simulink model "F429_OneADC"  (R2018b)
settings: Solver=FixedStepDiscrete  StartTime=0.0  StopTime=10.0  FixedStep=0.016  RelTol=1e-3  EnableMultiTasking=on
libraries: ADC_Lib x1, STM32_Config_Lib x1, TIMERS_Lib x1, USART_Lib x1
settings Model: Creator=reynaudp  LastModifiedBy=fenard1
settings DataIOCC: LimitDataPoints=on  SaveFormat=Array
settings OptimizationCC: DefaultParameterBehavior=Inlined  LifeSpan=1
settings DebuggingCC: UnderspecifiedInitializationDetection=Classic  MergeDetectMultiDrivingBlocksExec=none  SolverPrmCheckMsg=warning  UniqueDataStoreMsg=error  AllowSymbolicDim=off  StrictBusMsg=ErrorOnBusTreatedAsVector  SFUnexpectedBacktrackingDiag=warning  SFNoUnconditionalDefaultTransitionDiag=warning  SFExecutionAtInitializationDiag=none
settings HardwareCC: ProdBitPerPointer=32  ProdBitPerSizeT=32  ProdBitPerPtrDiffT=32  ProdLargestAtomicInteger=Integer  ProdWordSize=32  ProdHWDeviceType=STMicroelectronics->STM32 32-bit Cortex-M  TargetBitPerPointer=64  TargetBitPerSizeT=64  TargetBitPerPtrDiffT=64  TargetLongLongMode=on  TargetIntDivRoundTo=Zero  TargetEndianess=LittleEndian  TargetWordSize=64  TargetHWDeviceType=MATLAB Host  ProdEqTarget=off
settings ModelReferenceCC: PropagateSignalLabelsOutOfModel=off
settings SFSimCC: SimUseLocalCustomCode=off  CompileTimeRecursionLimit=0  EnableRuntimeRecursion=off  MATLABDynamicMemAlloc=off
settings RTWCC: SystemTargetFile=stm32.tlc  TemplateMakefile=stm32.tmf  Description=stm32 (Embedded Target)  RTWUseLocalCustomCode=off  IncludeHyperlinkInReport=on
settings CodeAppCC: IgnoreCustomStorageClasses=off  CustomSymbolStrType=$N$R$M  SimulinkBlockComments=off
settings STFCustomTargetCC: ParMdlRefBuildCompliant=on  IncludeMdlTerminateFcn=off  CombineOutputUpdateFcns=on  ERTCustomFileBanners=on  SupportComplex=off  SupportContinuousTime=off  SupportNonInlinedSFcns=off  RemoveResetFunc=on  MATLABClassNameForMDSCustomization=Simulink.SoftwareTarget.ERTCustomization  SystemTargetFile=stm32.tlc
settings ERTTargetCC: MultiwordLength=2048  CompOptLevelCompliant=off  ConcurrentExecutionCompliant=off  IncludeMdlTerminateFcn=off  SupportComplex=off  ModelStepFunctionPrototypeControlCompliant=off  CPPClassGenCompliant=off  UseToolchainInfoCompliant=off  ERTSrcFileBannerTemplate=sourceFileTemplate.cgt  ERTHdrFileBannerTemplate=sourceFileTemplate.cgt  ERTDataSrcFileTemplate=sourceFileTemplate.cgt  ERTDataHdrFileTemplate=sourceFileTemplate.cgt  ERTCustomFileTemplate=customRoutineProcess.tlc  ConvertIfToSwitch=off  SuppressUnreachableDefaultCases=off
settings ConfigComp: CovMetricSettings=dw  CovHtmlReporting=on  CovSaveCumulativeToWorkspaceVar=on  CovSaveSingleToWorkspaceVar=on  CovExternalEMLEnable=off  CovSFcnEnable=off

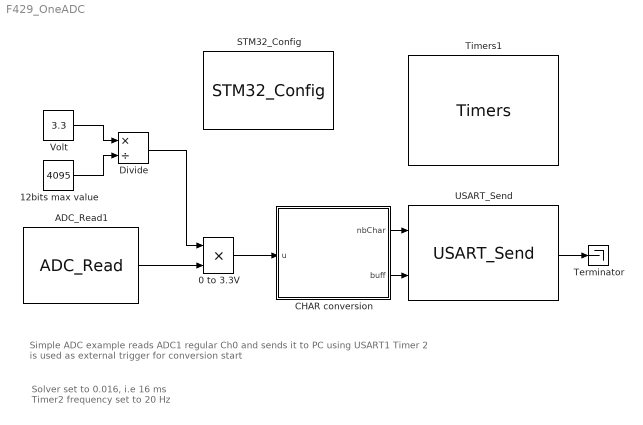
== system F429_OneADC ==
  note: Solver set to 0.016, i.e 16 ms
      | Timer2 frequency set to 20 Hz
  note: Simple ADC example reads ADC1 regular Ch0 and sends it to PC using USART1
      | Timer 2 is used as external trigger for conversion start
  0 to 3.3V : Product  RndMeth=Zero
  12bits max value : Constant  Value=4095
  ADC_Read1 : ADC_Lib/ADC_Read  ADC_Name=ADC1  ADC_Ch0=on  ADC_Ch1=off  ADC_Ch2=off  ADC_Ch3=off  ADC_Ch4=off  ADC_Ch5=off  ADC_Ch6=off  ADC_Ch7=off  ADC_Ch8=off  ADC_Ch9=off  ADC_Ch10=off  ADC_Ch11=off  ADC_Ch12=off  ADC_Ch13=off  ADC_Ch14=off  ADC_Ch15=off  ADC_Ch16=off  ADC_Ch17=off  ADC_Ch18=off  RgRk1=on  RgRk2=off  RgRk3=off  RgRk4=off  RgRk1_Ch=Ch0_r1  RgRk2_Ch=off  RgRk3_Ch=off  RgRk4_Ch=off  RgRk5=off  RgRk6=off  RgRk7=off  RgRk8=off  RgRk5_Ch=off  RgRk6_Ch=off  RgRk7_Ch=off  RgRk8_Ch=off  RgRk9=off  RgRk10=off  RgRk11=off  RgRk12=off  RgRk9_Ch=off  RgRk10_Ch=off  RgRk11_Ch=off  RgRk12_Ch=off  RgRk13=off  RgRk14=off  RgRk15=off  RgRk16=off  RgRk13_Ch=off  RgRk14_Ch=off  RgRk15_Ch=off  RgRk16_Ch=off  InjRk1=off  InjRk2=off  InjRk3=off  InjRk4=off  InjRk1_Ch=off  InjRk2_Ch=off  InjRk3_Ch=off  InjRk4_Ch=off  ADC_Trig=T2_TRGO  ADC_TrigEdge=Not used  DmaReq=off  DMA_Buffer=0  ItReq=off  AWD_Mode=NOT_USED  AWD_Ch=0  AWD_HThres=0  AWD_LThres=0  AWD_En_Int=off  AWD2_HThres=0  AWD2_LThres=0  AWD2_En_Int=off  AWD3_HThres=0  AWD3_LThres=0  AWD3_En_Int=off  EOC_SEQ=on  EOC_IT=off  JEOC_IT=off  AWD_IT=off  OVR_IT=off  CpltTrans=off  HalfTrans=off  ADC_RegNb=1  ADC_RegCh0=on  ADC_RegCh1=off  ADC_RegCh2=off  ADC_RegCh3=off  ADC_RegCh4=off  ADC_RegCh5=off  ADC_RegCh6=off  ADC_RegCh7=off  ADC_RegCh8=off  ADC_RegCh9=off  ADC_RegCh10=off  ADC_RegCh11=off  ADC_RegCh12=off  ADC_RegCh13=off  ADC_RegCh14=off  ADC_RegCh15=off  ADC_RegCh16=off  ADC_RegCh17=off  ADC_RegCh18=off  ADC_InjNb=0  ADC_InjCh0=off  ADC_InjCh1=off  ADC_InjCh2=off  ADC_InjCh3=off  ADC_InjCh4=off  ADC_InjCh5=off  ADC_InjCh6=off  ADC_InjCh7=off  ADC_InjCh8=off  ADC_InjCh9=off  ADC_InjCh10=off  ADC_InjCh11=off  ADC_InjCh12=off  ADC_InjCh13=off  ADC_InjCh14=off  ADC_InjCh15=off  ADC_InjCh16=off  ADC_InjCh17=off  ADC_InjCh18=off  NbADC=1  CurrentADC=ADC1
      settings: SourceProductName=Target Support Package - STM32 Adapter
  CHAR conversion : MATLAB Function  TreatAsAtomicUnit=on
      settings: AttributesFormatString=SystemSampleTime=%<SystemSampleTime>
  Divide : Product  Inputs=*/
  STM32_Config : STM32_Config_Lib/STM32_Config  Priority=0  Project_Path=.\  Config_File=F429_OneADC.ioc  MCU_Name=STM32F429ZITx
      settings: SourceProductName=Target Support Package - STM32 Adapter
  Terminator : Terminator
  Timers1 : TIMERS_Lib/Timers  currentTIM=TIM2  TIM_Name=TIM2  sysUsingTimer=on  TIM_APBClock=90000000  TIM_Set_Clk=on  TIM_Prescaler=449  TIM_Clock=200000.00  Variable_frequency=off  TIM_Set_OutFreq=off  TIM_ARR=10000  Output_frequency=20.00  Repetition_counter=0  TIM_Mode=Up  TIM_DMA=none  TIM_IRQ=on  TIM_IRQ_ONLY=on  TIM_UP=off  TIM_TRG=off  TIM_COM=off  TIM_BRK=off  NbTIM=1  CH1_enable=off  CH1N_enable=off  CH1_type=Unknown  CH1_DMA=off  CH1_int=off  CH1_edge=Rising  CH1_div=1  CH1_variable_duty=off  CH1_set_pulse=off  CH1_output_duty=0.00  CH1_pulse=0  CH2_enable=off  CH2N_enable=off  CH2_type=Unknown  CH2_DMA=off  CH2_int=off  CH2_edge=Rising  CH2_div=1  CH2_variable_duty=off  CH2_set_pulse=off  CH2_output_duty=0.00  CH2_pulse=0  CH3_enable=off  CH3N_enable=off  CH3_type=Unknown  CH3_DMA=off  CH3_int=off  CH3_edge=Rising  CH3_div=1  CH3_variable_duty=off  CH3_set_pulse=off  CH3_output_duty=0.00  CH3_pulse=0  CH4_enable=off  CH4N_enable=off  CH4_type=Unknown  CH4_DMA=off  CH4_int=off  CH4_edge=Rising  CH4_div=1  CH4_variable_duty=off  CH4_set_pulse=off  CH4_output_duty=0.00  CH4_pulse=0
      settings: SourceProductName=Target Support Package - STM32 Adapter
  USART_Send : USART_Lib/USART_Send  USART_name=USART1  Buff_size=128  nbUsart=1  usartMode=Asynchronous  usartDma_Rx=off  usartDma_Tx=off  usartIt=on
      settings: SourceProductName=Target Support Package - STM32 Adapter
  Volt : Constant  Value=3.3  OutDataTypeStr=single
  wires:
  Volt/1 -> Divide/1
  12bits max value/1 -> Divide/2
  Divide/1 -> 0 to 3.3V/1
  CHAR conversion/1(nbChar) -> USART_Send/1
  0 to 3.3V/1 -> CHAR conversion/1(u)
  CHAR conversion/2(buff) -> USART_Send/2
  ADC_Read1/1 -> 0 to 3.3V/2
  USART_Send/1 -> Terminator/1

== matlab function F429_OneADC/CHAR conversion ==
  data: u input; nbChar output uint16 size=1; buff output uint32 size=1
function [nbChar, buff] = convert(u)
if coder.target('Sfun')
    % Executing in MATLAB, Buff is null
    buff = uint32(0);
    nbChar = uint16(0);
else
    coder.cinclude('stdio.h');
    coder.cinclude('main.h');
    coder.cinclude('getBuffPtr.h');

    % Executing in the generated code.
    string = char(zeros(1,20));
    stringSize = uint16(size(string,2));
    stringFormat = char(['%08x-%5.2f V',13,10,0]);
    tick = uint32(0);
    tick = coder.ceval('HAL_GetTick');
    coder.ceval('snprintf',coder.wref(string),stringSize,coder.rref(stringFormat),tick,u);
    buff = coder.ceval('getBuffPtr',coder.rref(string));
    nbChar = stringSize;
end
end
